simulink model "eTRU_prototype_2_old_perhabs_with_measurements"  (R2021b)
settings: Solver=daessc  StartTime=0.0  StopTime=5000  MaxStep=1  RelTol=1e-2  AbsTol=1e-2
PostLoadFcn:
  | eTRU_prototype_2_init
InitFcn:
  | eTRU_prototype_2_start_sim
StartFcn:
  | tic
StopFcn:
  | toc
  | PlotSimResults
values from neighbouring files (symbols this model uses):
  AirFlow = [0 0 0 0 0 0 0 0 0 0;      2205 1950 1701 1679 1297 658 0 0 0 0;      2989 2767 2610 2594 2410 2343 2274 1771 0 0;      3704 3545 3432 3422 3307 3266 3216 2958 2888 2215]    [EC_FanData.m]
  ambient_temp = 20    [eTRU_prototype_2_start_sim.m]
  asm = block.DialogPrm(1).Data    [msfcn_StaticASM.m]
  box_start_temp = 20    [eTRU_prototype_2_start_sim.m]
  cargo_start_temp = box_start_temp    (= 20)    [eTRU_prototype_2_start_sim.m]
  Power = [5 5 5 5 5 5 5 5 5 5;      185 203 227 226 229 230 231 237 239 247;      420 442 458 461 496 509 522 528 530 538;      764 811 844 846 880 892 905 969 987 989]    [EC_FanData.m]
  Pressure = LimitValue(Pressure + LimitValue(Error/dvdP, -0.1, 0.1), obj.PressureMin/100000, obj.PressureMax/100000)    [CoolPropPyWrapper.m]    (also in EC_FanData.m = [0,127,217,225,316,349,383,559,607,865])
  Speed = [0,1840,2450,3060]    [EC_FanData.m]
libraries: fl_lib x109, nesl_utility x82, simulink_extras x13, SimscapeFluids_lib x4
(part 3 of 3)

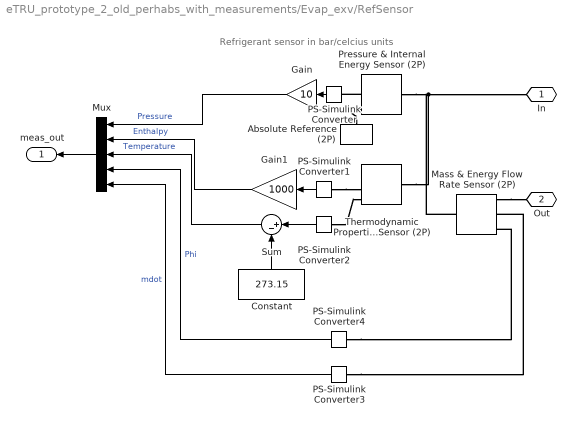
== system eTRU_prototype_2_old_perhabs_with_measurements/Evap_exv/RefSensor ==
  note: Refrigerant sensor in bar/celcius units
  Absolute Reference (2P) : fl_lib/Two-Phase Fluid/Elements/Absolute Reference (2P)
      settings: SourceProductBaseCode=SS
  Constant : Constant  Value=273.15
  Gain : Gain  Gain=10
  Gain1 : Gain  Gain=1000
  Mass & Energy Flow Rate Sensor (2P) : fl_lib/Two-Phase Fluid/Sensors/Mass & Energy Flow Rate Sensor (2P)
      settings: SourceProductBaseCode=SS  InternalSimscapePortConfiguration="{\"Bottom\":[],\"Left\":[{\"id\":\"A\",\"label\":\"A\",\"type\":\"foundation.two_phase_fluid.two_phase_fluid\"}],\"Right\":[{\"id\":\"B\",\"label\":\"B\",\"type\":\"foundation.two_phase_fluid.two_phase_fluid\"},{\"id\":\"M\",\"label\":\"M\",\"type\":\"output\"},{\"id\":\"PHI\",\"label\":\"Phi\",\"type\":\"output\"}],\"Top\":[]}"
  Mux : Mux  Inputs=5
  PS-Simulink Converter{,1..4} (5 alike) : nesl_utility/PS-Simulink Converter  PhysicalDomain=network_engine_domain  SubClassName=ps_output  LeftPortType=input  RightPortType=output  PseudoPeriodic=off  Frequencies=[]  Unit=inherit  AffineConversion=off
      settings: SourceProductBaseCode=PW,SS
  Pressure & Internal Energy Sensor (2P) : fl_lib/Two-Phase Fluid/Sensors/Pressure & Internal Energy Sensor (2P)
      settings: SourceProductBaseCode=SS  InternalSimscapePortConfiguration="{\"Bottom\":[],\"Left\":[{\"id\":\"A\",\"label\":\"A\",\"type\":\"foundation.two_phase_fluid.two_phase_fluid\"}],\"Right\":[{\"id\":\"B\",\"label\":\"B\",\"type\":\"foundation.two_phase_fluid.two_phase_fluid\"},{\"id\":\"P\",\"label\":\"P\",\"type\":\"output\"},{\"id\":\"U\",\"label\":\"U\",\"type\":\"output\"}],\"Top\":[]}"
  Sum : Sum  Inputs=|+-
  Thermodynamic Properties Sensor (2P) : fl_lib/Two-Phase Fluid/Sensors/Thermodynamic Properties Sensor (2P)
      settings: SourceProductBaseCode=SS  InternalSimscapePortConfiguration="{\"Bottom\":[],\"Left\":[{\"id\":\"A\",\"label\":\"A\",\"type\":\"foundation.two_phase_fluid.two_phase_fluid\"}],\"Right\":[{\"id\":\"T\",\"label\":\"T\",\"type\":\"output\"},{\"id\":\"H\",\"label\":\"h\",\"type\":\"output\"},{\"id\":\"V\",\"label\":\"v\",\"type\":\"output\"},{\"id\":\"S\",\"label\":\"s\",\"type\":\"output\"}],\"Top\":[]}"
  In : PMIOPort  Side=Left
  Out : PMIOPort  Port=2  Side=Right
  meas_out : Outport
  wires:
  Sum/1 -> Mux/3  "Temperature"
  PS-Simulink Converter1/1 -> Gain1/1
  Gain/1 -> Mux/1  "Pressure"
  PS-Simulink Converter2/1 -> Sum/1
  Mux/1 -> meas_out/1
  PS-Simulink Converter/1 -> Gain/1
  Constant/1 -> Sum/2
  Gain1/1 -> Mux/2  "Enthalpy"
  PS-Simulink Converter4/1 -> Mux/4  "Phi"
  PS-Simulink Converter3/1 -> Mux/5  "mdot"
  connections:
  Pressure & Internal Energy Sensor (2P)/LConn1 -- In/RConn1 -- Thermodynamic Properties Sensor (2P)/LConn1 -- Mass & Energy Flow Rate Sensor (2P)/LConn1
  PS-Simulink Converter1/LConn1 -- Thermodynamic Properties Sensor (2P)/RConn2
  Pressure & Internal Energy Sensor (2P)/RConn1 -- Absolute Reference (2P)/LConn1
  Pressure & Internal Energy Sensor (2P)/RConn2 -- PS-Simulink Converter/LConn1
  PS-Simulink Converter2/LConn1 -- Thermodynamic Properties Sensor (2P)/RConn1
  Mass & Energy Flow Rate Sensor (2P)/RConn1 -- Out/RConn1
  PS-Simulink Converter4/LConn1 -- Mass & Energy Flow Rate Sensor (2P)/RConn3
  PS-Simulink Converter3/LConn1 -- Mass & Energy Flow Rate Sensor (2P)/RConn2

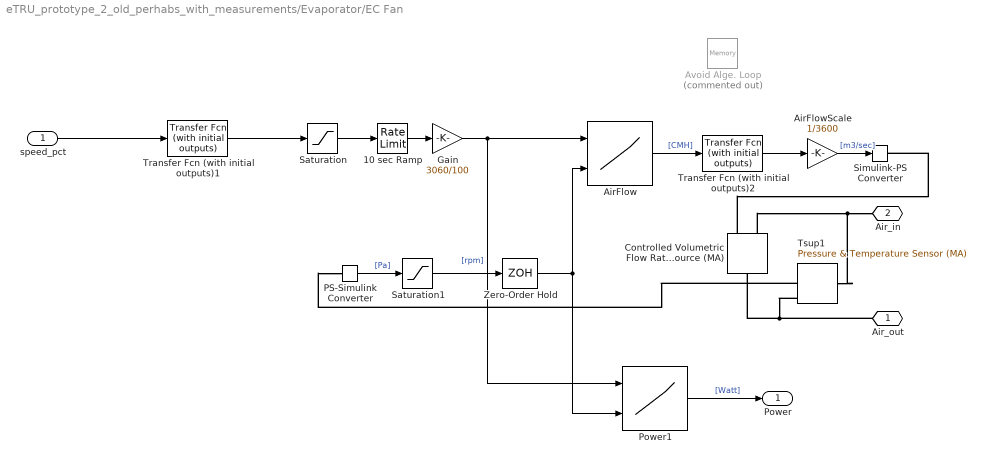
== system eTRU_prototype_2_old_perhabs_with_measurements/Evaporator/EC Fan ==
  speed_pct : Inport
  10 sec Ramp : RateLimiter  RisingSlewLimit=300  FallingSlewLimit=-300  SampleTimeMode=inherited
  AirFlow : Lookup_n-D  BreakpointsForDimension1=Speed  BreakpointsForDimension2=Pressure  BeginIndexSearchUsingPreviousIndexResult=on  Table=AirFlow  InternalRulePriority=Speed  RndMeth=Simplest  InputSameDT=on
      settings: InputPortMap=u0,u1
  AirFlowScale : Gain  Gain=1/3600
  Avoid Alge. Loop : Memory  Commented=on
  Controlled Volumetric Flow Rate Source (MA) : fl_lib/Moist Air/Sources/Controlled Volumetric Flow Rate Source (MA)  power_spec=foundation.enum.power_spec.isentropic  volumetric_flow_conditions=foundation.enum.volumetric_flow_conditions.actual  p_std=0.101325 MPa  T_std=20 degC  RH_std=0.65  area_A=0.2 m^2  area_B=0.2 m^2
      settings: SourceProductBaseCode=SS  InternalSimscapePortConfiguration="{\"Bottom\":[],\"Left\":[{\"id\":\"A\",\"label\":\"A\",\"type\":\"foundation.moist_air.moist_air\"},{\"id\":\"V\",\"label\":\"V\",\"type\":\"input\"}],\"Right\":[{\"id\":\"B\",\"label\":\"B\",\"type\":\"foundation.moist_air.moist_air\"}],\"Top\":[]}"
  Gain : Gain  Gain=3060/100
  PS-Simulink Converter : nesl_utility/PS-Simulink Converter  PhysicalDomain=network_engine_domain  SubClassName=ps_output  LeftPortType=input  RightPortType=output  PseudoPeriodic=off  Frequencies=[]  Unit=inherit  AffineConversion=off
      settings: SourceProductBaseCode=PW,SS
  Power1 : Lookup_n-D  BreakpointsForDimension1=Speed  BreakpointsForDimension2=Pressure  BeginIndexSearchUsingPreviousIndexResult=on  Table=Power  InternalRulePriority=Speed  RndMeth=Simplest  InputSameDT=on
      settings: InputPortMap=u0,u1
  Saturation : Saturate  UpperLimit=100  LowerLimit=0
  Saturation1 : Saturate  UpperLimit=865  LowerLimit=0
  Simulink-PS Converter : nesl_utility/Simulink-PS Converter  PhysicalDomain=network_engine_domain  SubClassName=ps_input  LeftPortType=input  RightPortType=output  PseudoPeriodic=off  Frequencies=[]  NoiseDistribution=none  NoiseParameters=[]  Unit=1  AffineConversion=off  FilteringAndDerivatives=provide  SimscapeFilterOrder=1  InputFilterTimeConstant=0.001  UdotUserProvided=0
      settings: SourceProductBaseCode=PW,SS
  Transfer Fcn (with initial outputs)1 : simulink_extras/Additional Linear/Transfer Fcn (with initial outputs)  N=[1]  D="[1  1]"  Y0=0  U0=0
  Transfer Fcn (with initial outputs)2 : simulink_extras/Additional Linear/Transfer Fcn (with initial outputs)  N=[1]  D="[1  1]"  Y0=0  U0=0
  Tsup1 : fl_lib/Moist Air/Sensors/Pressure & Temperature Sensor (MA)
      settings: SourceProductBaseCode=SS  InternalSimscapePortConfiguration="{\"Bottom\":[],\"Left\":[{\"id\":\"A\",\"label\":\"A\",\"type\":\"foundation.moist_air.moist_air\"}],\"Right\":[{\"id\":\"B\",\"label\":\"B\",\"type\":\"foundation.moist_air.moist_air\"},{\"id\":\"P\",\"label\":\"P\",\"type\":\"output\"},{\"id\":\"T\",\"label\":\"T\",\"type\":\"output\"}],\"Top\":[]}"
  Zero-Order Hold : ZeroOrderHold
  Air_out : PMIOPort  Side=Right
  Air_in : PMIOPort  Port=2  Side=Right
  Power : Outport
  wires:
  speed_pct/1 -> Transfer Fcn (with initial outputs)1/1
  Saturation/1 -> 10 sec Ramp/1
  10 sec Ramp/1 -> Gain/1
  Gain/1 -> Power1/1, AirFlow/1  "[rpm]"
  PS-Simulink Converter/1 -> Saturation1/1  "[Pa]"
  Saturation1/1 -> Zero-Order Hold/1
  Power1/1 -> Power/1  "[Watt]"
  AirFlowScale/1 -> Simulink-PS Converter/1  "[m3/sec]"
  Zero-Order Hold/1 -> AirFlow/2, Power1/2
  Transfer Fcn (with initial outputs)1/1 -> Saturation/1
  AirFlow/1 -> Transfer Fcn (with initial outputs)2/1  "[CMH]"
  Transfer Fcn (with initial outputs)2/1 -> AirFlowScale/1
  connections:
  Controlled Volumetric Flow Rate Source (MA)/LConn1 -- Tsup1/LConn1 -- Air_in/RConn1
  Controlled Volumetric Flow Rate Source (MA)/LConn2 -- Simulink-PS Converter/RConn1
  Air_out/RConn1 -- Tsup1/RConn1 -- Controlled Volumetric Flow Rate Source (MA)/RConn1
  Tsup1/RConn2 -- PS-Simulink Converter/LConn1

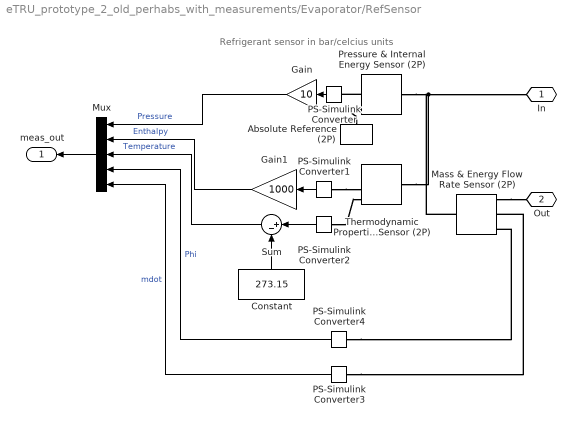
== system eTRU_prototype_2_old_perhabs_with_measurements/Evaporator/RefSensor ==
  note: Refrigerant sensor in bar/celcius units
  Absolute Reference (2P) : fl_lib/Two-Phase Fluid/Elements/Absolute Reference (2P)
      settings: SourceProductBaseCode=SS
  Constant : Constant  Value=273.15
  Gain : Gain  Gain=10
  Gain1 : Gain  Gain=1000
  Mass & Energy Flow Rate Sensor (2P) : fl_lib/Two-Phase Fluid/Sensors/Mass & Energy Flow Rate Sensor (2P)
      settings: SourceProductBaseCode=SS  InternalSimscapePortConfiguration="{\"Bottom\":[],\"Left\":[{\"id\":\"A\",\"label\":\"A\",\"type\":\"foundation.two_phase_fluid.two_phase_fluid\"}],\"Right\":[{\"id\":\"B\",\"label\":\"B\",\"type\":\"foundation.two_phase_fluid.two_phase_fluid\"},{\"id\":\"M\",\"label\":\"M\",\"type\":\"output\"},{\"id\":\"PHI\",\"label\":\"Phi\",\"type\":\"output\"}],\"Top\":[]}"
  Mux : Mux  Inputs=5
  PS-Simulink Converter{,1..4} (5 alike) : nesl_utility/PS-Simulink Converter  PhysicalDomain=network_engine_domain  SubClassName=ps_output  LeftPortType=input  RightPortType=output  PseudoPeriodic=off  Frequencies=[]  Unit=inherit  AffineConversion=off
      settings: SourceProductBaseCode=PW,SS
  Pressure & Internal Energy Sensor (2P) : fl_lib/Two-Phase Fluid/Sensors/Pressure & Internal Energy Sensor (2P)
      settings: SourceProductBaseCode=SS  InternalSimscapePortConfiguration="{\"Bottom\":[],\"Left\":[{\"id\":\"A\",\"label\":\"A\",\"type\":\"foundation.two_phase_fluid.two_phase_fluid\"}],\"Right\":[{\"id\":\"B\",\"label\":\"B\",\"type\":\"foundation.two_phase_fluid.two_phase_fluid\"},{\"id\":\"P\",\"label\":\"P\",\"type\":\"output\"},{\"id\":\"U\",\"label\":\"U\",\"type\":\"output\"}],\"Top\":[]}"
  Sum : Sum  Inputs=|+-
  Thermodynamic Properties Sensor (2P) : fl_lib/Two-Phase Fluid/Sensors/Thermodynamic Properties Sensor (2P)
      settings: SourceProductBaseCode=SS  InternalSimscapePortConfiguration="{\"Bottom\":[],\"Left\":[{\"id\":\"A\",\"label\":\"A\",\"type\":\"foundation.two_phase_fluid.two_phase_fluid\"}],\"Right\":[{\"id\":\"T\",\"label\":\"T\",\"type\":\"output\"},{\"id\":\"H\",\"label\":\"h\",\"type\":\"output\"},{\"id\":\"V\",\"label\":\"v\",\"type\":\"output\"},{\"id\":\"S\",\"label\":\"s\",\"type\":\"output\"}],\"Top\":[]}"
  In : PMIOPort  Side=Left
  Out : PMIOPort  Port=2  Side=Right
  meas_out : Outport
  wires:
  Sum/1 -> Mux/3  "Temperature"
  PS-Simulink Converter1/1 -> Gain1/1
  Gain/1 -> Mux/1  "Pressure"
  PS-Simulink Converter2/1 -> Sum/1
  Mux/1 -> meas_out/1
  PS-Simulink Converter/1 -> Gain/1
  Constant/1 -> Sum/2
  Gain1/1 -> Mux/2  "Enthalpy"
  PS-Simulink Converter4/1 -> Mux/4  "Phi"
  PS-Simulink Converter3/1 -> Mux/5  "mdot"
  connections:
  Pressure & Internal Energy Sensor (2P)/LConn1 -- In/RConn1 -- Thermodynamic Properties Sensor (2P)/LConn1 -- Mass & Energy Flow Rate Sensor (2P)/LConn1
  PS-Simulink Converter1/LConn1 -- Thermodynamic Properties Sensor (2P)/RConn2
  Pressure & Internal Energy Sensor (2P)/RConn1 -- Absolute Reference (2P)/LConn1
  Pressure & Internal Energy Sensor (2P)/RConn2 -- PS-Simulink Converter/LConn1
  PS-Simulink Converter2/LConn1 -- Thermodynamic Properties Sensor (2P)/RConn1
  Mass & Energy Flow Rate Sensor (2P)/RConn1 -- Out/RConn1
  PS-Simulink Converter4/LConn1 -- Mass & Energy Flow Rate Sensor (2P)/RConn3
  PS-Simulink Converter3/LConn1 -- Mass & Energy Flow Rate Sensor (2P)/RConn2

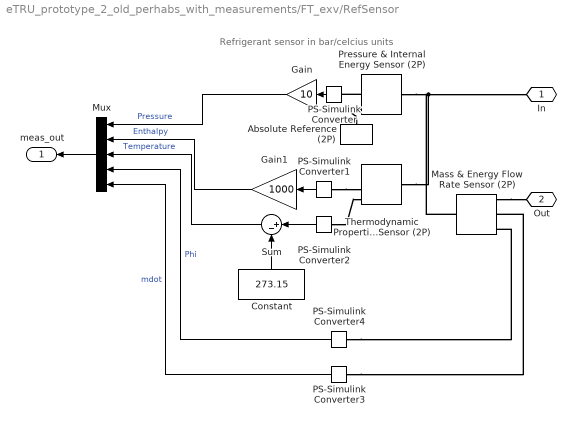
== system eTRU_prototype_2_old_perhabs_with_measurements/FT_exv/RefSensor ==
  note: Refrigerant sensor in bar/celcius units
  Absolute Reference (2P) : fl_lib/Two-Phase Fluid/Elements/Absolute Reference (2P)
      settings: SourceProductBaseCode=SS
  Constant : Constant  Value=273.15
  Gain : Gain  Gain=10
  Gain1 : Gain  Gain=1000
  Mass & Energy Flow Rate Sensor (2P) : fl_lib/Two-Phase Fluid/Sensors/Mass & Energy Flow Rate Sensor (2P)
      settings: SourceProductBaseCode=SS  InternalSimscapePortConfiguration="{\"Bottom\":[],\"Left\":[{\"id\":\"A\",\"label\":\"A\",\"type\":\"foundation.two_phase_fluid.two_phase_fluid\"}],\"Right\":[{\"id\":\"B\",\"label\":\"B\",\"type\":\"foundation.two_phase_fluid.two_phase_fluid\"},{\"id\":\"M\",\"label\":\"M\",\"type\":\"output\"},{\"id\":\"PHI\",\"label\":\"Phi\",\"type\":\"output\"}],\"Top\":[]}"
  Mux : Mux  Inputs=5
  PS-Simulink Converter{,1..4} (5 alike) : nesl_utility/PS-Simulink Converter  PhysicalDomain=network_engine_domain  SubClassName=ps_output  LeftPortType=input  RightPortType=output  PseudoPeriodic=off  Frequencies=[]  Unit=inherit  AffineConversion=off
      settings: SourceProductBaseCode=PW,SS
  Pressure & Internal Energy Sensor (2P) : fl_lib/Two-Phase Fluid/Sensors/Pressure & Internal Energy Sensor (2P)
      settings: SourceProductBaseCode=SS  InternalSimscapePortConfiguration="{\"Bottom\":[],\"Left\":[{\"id\":\"A\",\"label\":\"A\",\"type\":\"foundation.two_phase_fluid.two_phase_fluid\"}],\"Right\":[{\"id\":\"B\",\"label\":\"B\",\"type\":\"foundation.two_phase_fluid.two_phase_fluid\"},{\"id\":\"P\",\"label\":\"P\",\"type\":\"output\"},{\"id\":\"U\",\"label\":\"U\",\"type\":\"output\"}],\"Top\":[]}"
  Sum : Sum  Inputs=|+-
  Thermodynamic Properties Sensor (2P) : fl_lib/Two-Phase Fluid/Sensors/Thermodynamic Properties Sensor (2P)
      settings: SourceProductBaseCode=SS  InternalSimscapePortConfiguration="{\"Bottom\":[],\"Left\":[{\"id\":\"A\",\"label\":\"A\",\"type\":\"foundation.two_phase_fluid.two_phase_fluid\"}],\"Right\":[{\"id\":\"T\",\"label\":\"T\",\"type\":\"output\"},{\"id\":\"H\",\"label\":\"h\",\"type\":\"output\"},{\"id\":\"V\",\"label\":\"v\",\"type\":\"output\"},{\"id\":\"S\",\"label\":\"s\",\"type\":\"output\"}],\"Top\":[]}"
  In : PMIOPort  Side=Left
  Out : PMIOPort  Port=2  Side=Right
  meas_out : Outport
  wires:
  Sum/1 -> Mux/3  "Temperature"
  PS-Simulink Converter1/1 -> Gain1/1
  Gain/1 -> Mux/1  "Pressure"
  PS-Simulink Converter2/1 -> Sum/1
  Mux/1 -> meas_out/1
  PS-Simulink Converter/1 -> Gain/1
  Constant/1 -> Sum/2
  Gain1/1 -> Mux/2  "Enthalpy"
  PS-Simulink Converter4/1 -> Mux/4  "Phi"
  PS-Simulink Converter3/1 -> Mux/5  "mdot"
  connections:
  Pressure & Internal Energy Sensor (2P)/LConn1 -- In/RConn1 -- Thermodynamic Properties Sensor (2P)/LConn1 -- Mass & Energy Flow Rate Sensor (2P)/LConn1
  PS-Simulink Converter1/LConn1 -- Thermodynamic Properties Sensor (2P)/RConn2
  Pressure & Internal Energy Sensor (2P)/RConn1 -- Absolute Reference (2P)/LConn1
  Pressure & Internal Energy Sensor (2P)/RConn2 -- PS-Simulink Converter/LConn1
  PS-Simulink Converter2/LConn1 -- Thermodynamic Properties Sensor (2P)/RConn1
  Mass & Energy Flow Rate Sensor (2P)/RConn1 -- Out/RConn1
  PS-Simulink Converter4/LConn1 -- Mass & Energy Flow Rate Sensor (2P)/RConn3
  PS-Simulink Converter3/LConn1 -- Mass & Energy Flow Rate Sensor (2P)/RConn2

== system eTRU_prototype_2_old_perhabs_with_measurements/Flash tank/RefSensor ==
  note: Refrigerant sensor in bar/celcius units
  Absolute Reference (2P) : fl_lib/Two-Phase Fluid/Elements/Absolute Reference (2P)
      settings: SourceProductBaseCode=SS
  Constant : Constant  Value=273.15
  Gain : Gain  Gain=10
  Gain1 : Gain  Gain=1000
  Mass & Energy Flow Rate Sensor (2P) : fl_lib/Two-Phase Fluid/Sensors/Mass & Energy Flow Rate Sensor (2P)
      settings: SourceProductBaseCode=SS  InternalSimscapePortConfiguration="{\"Bottom\":[],\"Left\":[{\"id\":\"A\",\"label\":\"A\",\"type\":\"foundation.two_phase_fluid.two_phase_fluid\"}],\"Right\":[{\"id\":\"B\",\"label\":\"B\",\"type\":\"foundation.two_phase_fluid.two_phase_fluid\"},{\"id\":\"M\",\"label\":\"M\",\"type\":\"output\"},{\"id\":\"PHI\",\"label\":\"Phi\",\"type\":\"output\"}],\"Top\":[]}"
  Mux : Mux  Inputs=5
  PS-Simulink Converter{,1..4} (5 alike) : nesl_utility/PS-Simulink Converter  PhysicalDomain=network_engine_domain  SubClassName=ps_output  LeftPortType=input  RightPortType=output  PseudoPeriodic=off  Frequencies=[]  Unit=inherit  AffineConversion=off
      settings: SourceProductBaseCode=PW,SS
  Pressure & Internal Energy Sensor (2P) : fl_lib/Two-Phase Fluid/Sensors/Pressure & Internal Energy Sensor (2P)
      settings: SourceProductBaseCode=SS  InternalSimscapePortConfiguration="{\"Bottom\":[],\"Left\":[{\"id\":\"A\",\"label\":\"A\",\"type\":\"foundation.two_phase_fluid.two_phase_fluid\"}],\"Right\":[{\"id\":\"B\",\"label\":\"B\",\"type\":\"foundation.two_phase_fluid.two_phase_fluid\"},{\"id\":\"P\",\"label\":\"P\",\"type\":\"output\"},{\"id\":\"U\",\"label\":\"U\",\"type\":\"output\"}],\"Top\":[]}"
  Sum : Sum  Inputs=|+-
  Thermodynamic Properties Sensor (2P) : fl_lib/Two-Phase Fluid/Sensors/Thermodynamic Properties Sensor (2P)
      settings: SourceProductBaseCode=SS  InternalSimscapePortConfiguration="{\"Bottom\":[],\"Left\":[{\"id\":\"A\",\"label\":\"A\",\"type\":\"foundation.two_phase_fluid.two_phase_fluid\"}],\"Right\":[{\"id\":\"T\",\"label\":\"T\",\"type\":\"output\"},{\"id\":\"H\",\"label\":\"h\",\"type\":\"output\"},{\"id\":\"V\",\"label\":\"v\",\"type\":\"output\"},{\"id\":\"S\",\"label\":\"s\",\"type\":\"output\"}],\"Top\":[]}"
  In : PMIOPort  Side=Left
  Out : PMIOPort  Port=2  Side=Right
  meas_out : Outport
  wires:
  Sum/1 -> Mux/3  "Temperature"
  PS-Simulink Converter1/1 -> Gain1/1
  Gain/1 -> Mux/1  "Pressure"
  PS-Simulink Converter2/1 -> Sum/1
  Mux/1 -> meas_out/1
  PS-Simulink Converter/1 -> Gain/1
  Constant/1 -> Sum/2
  Gain1/1 -> Mux/2  "Enthalpy"
  PS-Simulink Converter4/1 -> Mux/4  "Phi"
  PS-Simulink Converter3/1 -> Mux/5  "mdot"
  connections:
  Pressure & Internal Energy Sensor (2P)/LConn1 -- In/RConn1 -- Thermodynamic Properties Sensor (2P)/LConn1 -- Mass & Energy Flow Rate Sensor (2P)/LConn1
  PS-Simulink Converter1/LConn1 -- Thermodynamic Properties Sensor (2P)/RConn2
  Pressure & Internal Energy Sensor (2P)/RConn1 -- Absolute Reference (2P)/LConn1
  Pressure & Internal Energy Sensor (2P)/RConn2 -- PS-Simulink Converter/LConn1
  PS-Simulink Converter2/LConn1 -- Thermodynamic Properties Sensor (2P)/RConn1
  Mass & Energy Flow Rate Sensor (2P)/RConn1 -- Out/RConn1
  PS-Simulink Converter4/LConn1 -- Mass & Energy Flow Rate Sensor (2P)/RConn3
  PS-Simulink Converter3/LConn1 -- Mass & Energy Flow Rate Sensor (2P)/RConn2

== system eTRU_prototype_2_old_perhabs_with_measurements/Flash tank/RefSensor1 ==
  note: Refrigerant sensor in bar/celcius units
  Absolute Reference (2P) : fl_lib/Two-Phase Fluid/Elements/Absolute Reference (2P)
      settings: SourceProductBaseCode=SS
  Constant : Constant  Value=273.15
  Gain : Gain  Gain=10
  Gain1 : Gain  Gain=1000
  Mass & Energy Flow Rate Sensor (2P) : fl_lib/Two-Phase Fluid/Sensors/Mass & Energy Flow Rate Sensor (2P)
      settings: SourceProductBaseCode=SS  InternalSimscapePortConfiguration="{\"Bottom\":[],\"Left\":[{\"id\":\"A\",\"label\":\"A\",\"type\":\"foundation.two_phase_fluid.two_phase_fluid\"}],\"Right\":[{\"id\":\"B\",\"label\":\"B\",\"type\":\"foundation.two_phase_fluid.two_phase_fluid\"},{\"id\":\"M\",\"label\":\"M\",\"type\":\"output\"},{\"id\":\"PHI\",\"label\":\"Phi\",\"type\":\"output\"}],\"Top\":[]}"
  Mux : Mux  Inputs=5
  PS-Simulink Converter{,1..4} (5 alike) : nesl_utility/PS-Simulink Converter  PhysicalDomain=network_engine_domain  SubClassName=ps_output  LeftPortType=input  RightPortType=output  PseudoPeriodic=off  Frequencies=[]  Unit=inherit  AffineConversion=off
      settings: SourceProductBaseCode=PW,SS
  Pressure & Internal Energy Sensor (2P) : fl_lib/Two-Phase Fluid/Sensors/Pressure & Internal Energy Sensor (2P)
      settings: SourceProductBaseCode=SS  InternalSimscapePortConfiguration="{\"Bottom\":[],\"Left\":[{\"id\":\"A\",\"label\":\"A\",\"type\":\"foundation.two_phase_fluid.two_phase_fluid\"}],\"Right\":[{\"id\":\"B\",\"label\":\"B\",\"type\":\"foundation.two_phase_fluid.two_phase_fluid\"},{\"id\":\"P\",\"label\":\"P\",\"type\":\"output\"},{\"id\":\"U\",\"label\":\"U\",\"type\":\"output\"}],\"Top\":[]}"
  Sum : Sum  Inputs=|+-
  Thermodynamic Properties Sensor (2P) : fl_lib/Two-Phase Fluid/Sensors/Thermodynamic Properties Sensor (2P)
      settings: SourceProductBaseCode=SS  InternalSimscapePortConfiguration="{\"Bottom\":[],\"Left\":[{\"id\":\"A\",\"label\":\"A\",\"type\":\"foundation.two_phase_fluid.two_phase_fluid\"}],\"Right\":[{\"id\":\"T\",\"label\":\"T\",\"type\":\"output\"},{\"id\":\"H\",\"label\":\"h\",\"type\":\"output\"},{\"id\":\"V\",\"label\":\"v\",\"type\":\"output\"},{\"id\":\"S\",\"label\":\"s\",\"type\":\"output\"}],\"Top\":[]}"
  In : PMIOPort  Side=Left
  Out : PMIOPort  Port=2  Side=Right
  meas_out : Outport
  wires:
  Sum/1 -> Mux/3  "Temperature"
  PS-Simulink Converter1/1 -> Gain1/1
  Gain/1 -> Mux/1  "Pressure"
  PS-Simulink Converter2/1 -> Sum/1
  Mux/1 -> meas_out/1
  PS-Simulink Converter/1 -> Gain/1
  Constant/1 -> Sum/2
  Gain1/1 -> Mux/2  "Enthalpy"
  PS-Simulink Converter4/1 -> Mux/4  "Phi"
  PS-Simulink Converter3/1 -> Mux/5  "mdot"
  connections:
  Pressure & Internal Energy Sensor (2P)/LConn1 -- In/RConn1 -- Thermodynamic Properties Sensor (2P)/LConn1 -- Mass & Energy Flow Rate Sensor (2P)/LConn1
  PS-Simulink Converter1/LConn1 -- Thermodynamic Properties Sensor (2P)/RConn2
  Pressure & Internal Energy Sensor (2P)/RConn1 -- Absolute Reference (2P)/LConn1
  Pressure & Internal Energy Sensor (2P)/RConn2 -- PS-Simulink Converter/LConn1
  PS-Simulink Converter2/LConn1 -- Thermodynamic Properties Sensor (2P)/RConn1
  Mass & Energy Flow Rate Sensor (2P)/RConn1 -- Out/RConn1
  PS-Simulink Converter4/LConn1 -- Mass & Energy Flow Rate Sensor (2P)/RConn3
  PS-Simulink Converter3/LConn1 -- Mass & Energy Flow Rate Sensor (2P)/RConn2

== system eTRU_prototype_2_old_perhabs_with_measurements/two_stage_compressor/COM1 in ==
  note: Refrigerant sensor in bar/celcius units
  Absolute Reference (2P) : fl_lib/Two-Phase Fluid/Elements/Absolute Reference (2P)
      settings: SourceProductBaseCode=SS
  Constant : Constant  Value=273.15
  Gain : Gain  Gain=10
  Gain1 : Gain  Gain=1000
  Mass & Energy Flow Rate Sensor (2P) : fl_lib/Two-Phase Fluid/Sensors/Mass & Energy Flow Rate Sensor (2P)
      settings: SourceProductBaseCode=SS  InternalSimscapePortConfiguration="{\"Bottom\":[],\"Left\":[{\"id\":\"A\",\"label\":\"A\",\"type\":\"foundation.two_phase_fluid.two_phase_fluid\"}],\"Right\":[{\"id\":\"B\",\"label\":\"B\",\"type\":\"foundation.two_phase_fluid.two_phase_fluid\"},{\"id\":\"M\",\"label\":\"M\",\"type\":\"output\"},{\"id\":\"PHI\",\"label\":\"Phi\",\"type\":\"output\"}],\"Top\":[]}"
  Mux : Mux  Inputs=5
  PS-Simulink Converter{,1..4} (5 alike) : nesl_utility/PS-Simulink Converter  PhysicalDomain=network_engine_domain  SubClassName=ps_output  LeftPortType=input  RightPortType=output  PseudoPeriodic=off  Frequencies=[]  Unit=inherit  AffineConversion=off
      settings: SourceProductBaseCode=PW,SS
  Pressure & Internal Energy Sensor (2P) : fl_lib/Two-Phase Fluid/Sensors/Pressure & Internal Energy Sensor (2P)
      settings: SourceProductBaseCode=SS  InternalSimscapePortConfiguration="{\"Bottom\":[],\"Left\":[{\"id\":\"A\",\"label\":\"A\",\"type\":\"foundation.two_phase_fluid.two_phase_fluid\"}],\"Right\":[{\"id\":\"B\",\"label\":\"B\",\"type\":\"foundation.two_phase_fluid.two_phase_fluid\"},{\"id\":\"P\",\"label\":\"P\",\"type\":\"output\"},{\"id\":\"U\",\"label\":\"U\",\"type\":\"output\"}],\"Top\":[]}"
  Sum : Sum  Inputs=|+-
  Thermodynamic Properties Sensor (2P) : fl_lib/Two-Phase Fluid/Sensors/Thermodynamic Properties Sensor (2P)
      settings: SourceProductBaseCode=SS  InternalSimscapePortConfiguration="{\"Bottom\":[],\"Left\":[{\"id\":\"A\",\"label\":\"A\",\"type\":\"foundation.two_phase_fluid.two_phase_fluid\"}],\"Right\":[{\"id\":\"T\",\"label\":\"T\",\"type\":\"output\"},{\"id\":\"H\",\"label\":\"h\",\"type\":\"output\"},{\"id\":\"V\",\"label\":\"v\",\"type\":\"output\"},{\"id\":\"S\",\"label\":\"s\",\"type\":\"output\"}],\"Top\":[]}"
  In : PMIOPort  Side=Left
  Out : PMIOPort  Port=2  Side=Right
  meas_out : Outport
  wires:
  Sum/1 -> Mux/3  "Temperature"
  PS-Simulink Converter1/1 -> Gain1/1
  Gain/1 -> Mux/1  "Pressure"
  PS-Simulink Converter2/1 -> Sum/1
  Mux/1 -> meas_out/1
  PS-Simulink Converter/1 -> Gain/1
  Constant/1 -> Sum/2
  Gain1/1 -> Mux/2  "Enthalpy"
  PS-Simulink Converter4/1 -> Mux/4  "Phi"
  PS-Simulink Converter3/1 -> Mux/5  "mdot"
  connections:
  Pressure & Internal Energy Sensor (2P)/LConn1 -- Mass & Energy Flow Rate Sensor (2P)/LConn1 -- Thermodynamic Properties Sensor (2P)/LConn1 -- In/RConn1
  PS-Simulink Converter1/LConn1 -- Thermodynamic Properties Sensor (2P)/RConn2
  Pressure & Internal Energy Sensor (2P)/RConn1 -- Absolute Reference (2P)/LConn1
  Pressure & Internal Energy Sensor (2P)/RConn2 -- PS-Simulink Converter/LConn1
  PS-Simulink Converter2/LConn1 -- Thermodynamic Properties Sensor (2P)/RConn1
  Mass & Energy Flow Rate Sensor (2P)/RConn1 -- Out/RConn1
  PS-Simulink Converter4/LConn1 -- Mass & Energy Flow Rate Sensor (2P)/RConn3
  PS-Simulink Converter3/LConn1 -- Mass & Energy Flow Rate Sensor (2P)/RConn2

== system eTRU_prototype_2_old_perhabs_with_measurements/two_stage_compressor/COM1 out ==
  note: Refrigerant sensor in bar/celcius units
  Absolute Reference (2P) : fl_lib/Two-Phase Fluid/Elements/Absolute Reference (2P)
      settings: SourceProductBaseCode=SS
  Constant : Constant  Value=273.15
  Gain : Gain  Gain=10
  Gain1 : Gain  Gain=1000
  Mass & Energy Flow Rate Sensor (2P) : fl_lib/Two-Phase Fluid/Sensors/Mass & Energy Flow Rate Sensor (2P)
      settings: SourceProductBaseCode=SS  InternalSimscapePortConfiguration="{\"Bottom\":[],\"Left\":[{\"id\":\"A\",\"label\":\"A\",\"type\":\"foundation.two_phase_fluid.two_phase_fluid\"}],\"Right\":[{\"id\":\"B\",\"label\":\"B\",\"type\":\"foundation.two_phase_fluid.two_phase_fluid\"},{\"id\":\"M\",\"label\":\"M\",\"type\":\"output\"},{\"id\":\"PHI\",\"label\":\"Phi\",\"type\":\"output\"}],\"Top\":[]}"
  Mux : Mux  Inputs=5
  PS-Simulink Converter{,1..4} (5 alike) : nesl_utility/PS-Simulink Converter  PhysicalDomain=network_engine_domain  SubClassName=ps_output  LeftPortType=input  RightPortType=output  PseudoPeriodic=off  Frequencies=[]  Unit=inherit  AffineConversion=off
      settings: SourceProductBaseCode=PW,SS
  Pressure & Internal Energy Sensor (2P) : fl_lib/Two-Phase Fluid/Sensors/Pressure & Internal Energy Sensor (2P)
      settings: SourceProductBaseCode=SS  InternalSimscapePortConfiguration="{\"Bottom\":[],\"Left\":[{\"id\":\"A\",\"label\":\"A\",\"type\":\"foundation.two_phase_fluid.two_phase_fluid\"}],\"Right\":[{\"id\":\"B\",\"label\":\"B\",\"type\":\"foundation.two_phase_fluid.two_phase_fluid\"},{\"id\":\"P\",\"label\":\"P\",\"type\":\"output\"},{\"id\":\"U\",\"label\":\"U\",\"type\":\"output\"}],\"Top\":[]}"
  Sum : Sum  Inputs=|+-
  Thermodynamic Properties Sensor (2P) : fl_lib/Two-Phase Fluid/Sensors/Thermodynamic Properties Sensor (2P)
      settings: SourceProductBaseCode=SS  InternalSimscapePortConfiguration="{\"Bottom\":[],\"Left\":[{\"id\":\"A\",\"label\":\"A\",\"type\":\"foundation.two_phase_fluid.two_phase_fluid\"}],\"Right\":[{\"id\":\"T\",\"label\":\"T\",\"type\":\"output\"},{\"id\":\"H\",\"label\":\"h\",\"type\":\"output\"},{\"id\":\"V\",\"label\":\"v\",\"type\":\"output\"},{\"id\":\"S\",\"label\":\"s\",\"type\":\"output\"}],\"Top\":[]}"
  In : PMIOPort  Side=Left
  Out : PMIOPort  Port=2  Side=Right
  meas_out : Outport
  wires:
  Sum/1 -> Mux/3  "Temperature"
  PS-Simulink Converter1/1 -> Gain1/1
  Gain/1 -> Mux/1  "Pressure"
  PS-Simulink Converter2/1 -> Sum/1
  Mux/1 -> meas_out/1
  PS-Simulink Converter/1 -> Gain/1
  Constant/1 -> Sum/2
  Gain1/1 -> Mux/2  "Enthalpy"
  PS-Simulink Converter4/1 -> Mux/4  "Phi"
  PS-Simulink Converter3/1 -> Mux/5  "mdot"
  connections:
  Pressure & Internal Energy Sensor (2P)/LConn1 -- Mass & Energy Flow Rate Sensor (2P)/LConn1 -- Thermodynamic Properties Sensor (2P)/LConn1 -- In/RConn1
  PS-Simulink Converter1/LConn1 -- Thermodynamic Properties Sensor (2P)/RConn2
  Pressure & Internal Energy Sensor (2P)/RConn1 -- Absolute Reference (2P)/LConn1
  Pressure & Internal Energy Sensor (2P)/RConn2 -- PS-Simulink Converter/LConn1
  PS-Simulink Converter2/LConn1 -- Thermodynamic Properties Sensor (2P)/RConn1
  Mass & Energy Flow Rate Sensor (2P)/RConn1 -- Out/RConn1
  PS-Simulink Converter4/LConn1 -- Mass & Energy Flow Rate Sensor (2P)/RConn3
  PS-Simulink Converter3/LConn1 -- Mass & Energy Flow Rate Sensor (2P)/RConn2

== system eTRU_prototype_2_old_perhabs_with_measurements/two_stage_compressor/COM2 in ==
  note: Refrigerant sensor in bar/celcius units
  Absolute Reference (2P) : fl_lib/Two-Phase Fluid/Elements/Absolute Reference (2P)
      settings: SourceProductBaseCode=SS
  Constant : Constant  Value=273.15
  Gain : Gain  Gain=10
  Gain1 : Gain  Gain=1000
  Mass & Energy Flow Rate Sensor (2P) : fl_lib/Two-Phase Fluid/Sensors/Mass & Energy Flow Rate Sensor (2P)
      settings: SourceProductBaseCode=SS  InternalSimscapePortConfiguration="{\"Bottom\":[],\"Left\":[{\"id\":\"A\",\"label\":\"A\",\"type\":\"foundation.two_phase_fluid.two_phase_fluid\"}],\"Right\":[{\"id\":\"B\",\"label\":\"B\",\"type\":\"foundation.two_phase_fluid.two_phase_fluid\"},{\"id\":\"M\",\"label\":\"M\",\"type\":\"output\"},{\"id\":\"PHI\",\"label\":\"Phi\",\"type\":\"output\"}],\"Top\":[]}"
  Mux : Mux  Inputs=5
  PS-Simulink Converter{,1..4} (5 alike) : nesl_utility/PS-Simulink Converter  PhysicalDomain=network_engine_domain  SubClassName=ps_output  LeftPortType=input  RightPortType=output  PseudoPeriodic=off  Frequencies=[]  Unit=inherit  AffineConversion=off
      settings: SourceProductBaseCode=PW,SS
  Pressure & Internal Energy Sensor (2P) : fl_lib/Two-Phase Fluid/Sensors/Pressure & Internal Energy Sensor (2P)
      settings: SourceProductBaseCode=SS  InternalSimscapePortConfiguration="{\"Bottom\":[],\"Left\":[{\"id\":\"A\",\"label\":\"A\",\"type\":\"foundation.two_phase_fluid.two_phase_fluid\"}],\"Right\":[{\"id\":\"B\",\"label\":\"B\",\"type\":\"foundation.two_phase_fluid.two_phase_fluid\"},{\"id\":\"P\",\"label\":\"P\",\"type\":\"output\"},{\"id\":\"U\",\"label\":\"U\",\"type\":\"output\"}],\"Top\":[]}"
  Sum : Sum  Inputs=|+-
  Thermodynamic Properties Sensor (2P) : fl_lib/Two-Phase Fluid/Sensors/Thermodynamic Properties Sensor (2P)
      settings: SourceProductBaseCode=SS  InternalSimscapePortConfiguration="{\"Bottom\":[],\"Left\":[{\"id\":\"A\",\"label\":\"A\",\"type\":\"foundation.two_phase_fluid.two_phase_fluid\"}],\"Right\":[{\"id\":\"T\",\"label\":\"T\",\"type\":\"output\"},{\"id\":\"H\",\"label\":\"h\",\"type\":\"output\"},{\"id\":\"V\",\"label\":\"v\",\"type\":\"output\"},{\"id\":\"S\",\"label\":\"s\",\"type\":\"output\"}],\"Top\":[]}"
  In : PMIOPort  Side=Left
  Out : PMIOPort  Port=2  Side=Right
  meas_out : Outport
  wires:
  Sum/1 -> Mux/3  "Temperature"
  PS-Simulink Converter1/1 -> Gain1/1
  Gain/1 -> Mux/1  "Pressure"
  PS-Simulink Converter2/1 -> Sum/1
  Mux/1 -> meas_out/1
  PS-Simulink Converter/1 -> Gain/1
  Constant/1 -> Sum/2
  Gain1/1 -> Mux/2  "Enthalpy"
  PS-Simulink Converter4/1 -> Mux/4  "Phi"
  PS-Simulink Converter3/1 -> Mux/5  "mdot"
  connections:
  Pressure & Internal Energy Sensor (2P)/LConn1 -- Mass & Energy Flow Rate Sensor (2P)/LConn1 -- Thermodynamic Properties Sensor (2P)/LConn1 -- In/RConn1
  PS-Simulink Converter1/LConn1 -- Thermodynamic Properties Sensor (2P)/RConn2
  Pressure & Internal Energy Sensor (2P)/RConn1 -- Absolute Reference (2P)/LConn1
  Pressure & Internal Energy Sensor (2P)/RConn2 -- PS-Simulink Converter/LConn1
  PS-Simulink Converter2/LConn1 -- Thermodynamic Properties Sensor (2P)/RConn1
  Mass & Energy Flow Rate Sensor (2P)/RConn1 -- Out/RConn1
  PS-Simulink Converter4/LConn1 -- Mass & Energy Flow Rate Sensor (2P)/RConn3
  PS-Simulink Converter3/LConn1 -- Mass & Energy Flow Rate Sensor (2P)/RConn2

== system eTRU_prototype_2_old_perhabs_with_measurements/two_stage_compressor/Discharge ==
  note: Refrigerant sensor in bar/celcius units
  Absolute Reference (2P) : fl_lib/Two-Phase Fluid/Elements/Absolute Reference (2P)
      settings: SourceProductBaseCode=SS
  Constant : Constant  Value=273.15
  Gain : Gain  Gain=10
  Gain1 : Gain  Gain=1000
  Mass & Energy Flow Rate Sensor (2P) : fl_lib/Two-Phase Fluid/Sensors/Mass & Energy Flow Rate Sensor (2P)
      settings: SourceProductBaseCode=SS  InternalSimscapePortConfiguration="{\"Bottom\":[],\"Left\":[{\"id\":\"A\",\"label\":\"A\",\"type\":\"foundation.two_phase_fluid.two_phase_fluid\"}],\"Right\":[{\"id\":\"B\",\"label\":\"B\",\"type\":\"foundation.two_phase_fluid.two_phase_fluid\"},{\"id\":\"M\",\"label\":\"M\",\"type\":\"output\"},{\"id\":\"PHI\",\"label\":\"Phi\",\"type\":\"output\"}],\"Top\":[]}"
  Mux : Mux  Inputs=5
  PS-Simulink Converter{,1..4} (5 alike) : nesl_utility/PS-Simulink Converter  PhysicalDomain=network_engine_domain  SubClassName=ps_output  LeftPortType=input  RightPortType=output  PseudoPeriodic=off  Frequencies=[]  Unit=inherit  AffineConversion=off
      settings: SourceProductBaseCode=PW,SS
  Pressure & Internal Energy Sensor (2P) : fl_lib/Two-Phase Fluid/Sensors/Pressure & Internal Energy Sensor (2P)
      settings: SourceProductBaseCode=SS  InternalSimscapePortConfiguration="{\"Bottom\":[],\"Left\":[{\"id\":\"A\",\"label\":\"A\",\"type\":\"foundation.two_phase_fluid.two_phase_fluid\"}],\"Right\":[{\"id\":\"B\",\"label\":\"B\",\"type\":\"foundation.two_phase_fluid.two_phase_fluid\"},{\"id\":\"P\",\"label\":\"P\",\"type\":\"output\"},{\"id\":\"U\",\"label\":\"U\",\"type\":\"output\"}],\"Top\":[]}"
  Sum : Sum  Inputs=|+-
  Thermodynamic Properties Sensor (2P) : fl_lib/Two-Phase Fluid/Sensors/Thermodynamic Properties Sensor (2P)
      settings: SourceProductBaseCode=SS  InternalSimscapePortConfiguration="{\"Bottom\":[],\"Left\":[{\"id\":\"A\",\"label\":\"A\",\"type\":\"foundation.two_phase_fluid.two_phase_fluid\"}],\"Right\":[{\"id\":\"T\",\"label\":\"T\",\"type\":\"output\"},{\"id\":\"H\",\"label\":\"h\",\"type\":\"output\"},{\"id\":\"V\",\"label\":\"v\",\"type\":\"output\"},{\"id\":\"S\",\"label\":\"s\",\"type\":\"output\"}],\"Top\":[]}"
  In : PMIOPort  Side=Left
  Out : PMIOPort  Port=2  Side=Right
  meas_out : Outport
  wires:
  Sum/1 -> Mux/3  "Temperature"
  PS-Simulink Converter1/1 -> Gain1/1
  Gain/1 -> Mux/1  "Pressure"
  PS-Simulink Converter2/1 -> Sum/1
  Mux/1 -> meas_out/1
  PS-Simulink Converter/1 -> Gain/1
  Constant/1 -> Sum/2
  Gain1/1 -> Mux/2  "Enthalpy"
  PS-Simulink Converter4/1 -> Mux/4  "Phi"
  PS-Simulink Converter3/1 -> Mux/5  "mdot"
  connections:
  Pressure & Internal Energy Sensor (2P)/LConn1 -- Mass & Energy Flow Rate Sensor (2P)/LConn1 -- Thermodynamic Properties Sensor (2P)/LConn1 -- In/RConn1
  PS-Simulink Converter1/LConn1 -- Thermodynamic Properties Sensor (2P)/RConn2
  Pressure & Internal Energy Sensor (2P)/RConn1 -- Absolute Reference (2P)/LConn1
  Pressure & Internal Energy Sensor (2P)/RConn2 -- PS-Simulink Converter/LConn1
  PS-Simulink Converter2/LConn1 -- Thermodynamic Properties Sensor (2P)/RConn1
  Mass & Energy Flow Rate Sensor (2P)/RConn1 -- Out/RConn1
  PS-Simulink Converter4/LConn1 -- Mass & Energy Flow Rate Sensor (2P)/RConn3
  PS-Simulink Converter3/LConn1 -- Mass & Energy Flow Rate Sensor (2P)/RConn2

== system eTRU_prototype_2_old_perhabs_with_measurements/two_stage_compressor/MotorLossModel ==
  MotorLoad[kW] : Inport
  cpr_speed_pct : Inport  Port=2
  10 sec Ramp : RateLimiter  RisingSlewLimit=5  FallingSlewLimit=-5  SampleTimeMode=inherited
  AvoidDivBy0 : Saturate  UpperLimit=100  LowerLimit=10
  Divide : Product  Inputs=*/
  Gain : Gain  Gain=1000
  Gain2 : Gain  Gain=50/100*2*pi/asm.nom.Zpp
  Gain3 : Gain  Gain=50/100
  Gain4 : Gain  Gain=2*pi
  Level-2 MATLAB S-Function : M-S-Function  FunctionName=msfcn_StaticASM  Parameters=asm
  U/f : Fcn  Expr=(asm.nom.UfGain*u(1) + asm.nom.UfOffset)/1.5/sqrt(2)
  Iphase[Arms] : Outport
  wires:
  Gain2/1 -> Divide/2  "Wmech [rad/se]"
  U/f/1 -> Level-2 MATLAB S-Function/1  "Ufase [Vrms]"
  MotorLoad[kW]/1 -> Gain/1  "[kW]"
  10 sec Ramp/1 -> Gain3/1
  Gain/1 -> Divide/1  "[W]"
  Gain4/1 -> U/f/1  "F [rad/sec]"
  Gain3/1 -> Gain4/1, Level-2 MATLAB S-Function/2  "F [Hz]"
  AvoidDivBy0/1 -> Gain2/1
  Divide/1 -> Level-2 MATLAB S-Function/3  "Torque[Nm]"
  Level-2 MATLAB S-Function/1 -> Iphase[Arms]/1  "Iphase[Arms]"
  cpr_speed_pct/1 -> 10 sec Ramp/1, AvoidDivBy0/1
